simulink model "reaktor_m"  (R2016a)
settings: Solver=VariableStepAuto  StartTime=0.0  StopTime=400  RelTol=1e-3
undefined symbols (not defined in the file): AUXCO_0, B_t, C_0, linsys_matlab, P_cor0, ro_ex0, T_aves0, T_cl0, T_clp0, T_f10, T_f20, T_f30, T_hl0, T_hlp0, T_lp0, T_mo10, T_mo20, T_mo30, T_mo40, T_mo50, T_mo60, T_po0, T_set0, T_up0
settings Model: Creator=Użytkownik  LastModifiedBy=Michal Chruscinski
settings GRTTargetCC: GeneratePreprocessorConditionals=Use local settings

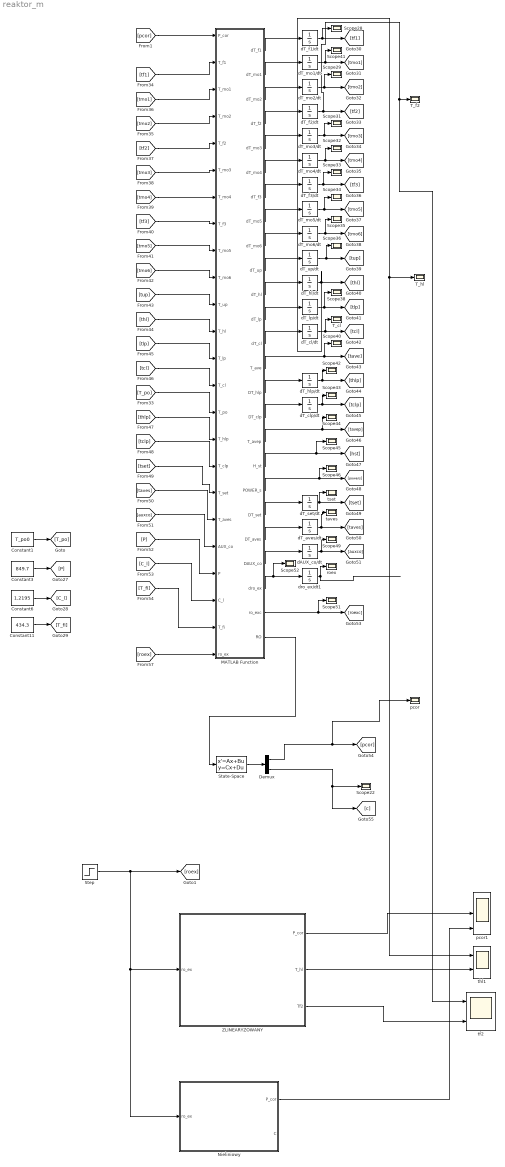
== system reaktor_m ==
  Constant1 : Constant  Value=T_po0
  Constant11 : Constant  Value=434.3
  Constant3 : Constant  Value=849.7
  Constant6 : Constant  Value=1.2195
  Demux : Demux  Outputs=2
  MATLAB Function : MATLAB Function  TreatAsAtomicUnit=on
  Nieliniowy : Subsystem
  Scope{22,28..29,31..36,38,40..46,49,51..52} (20 alike) : Scope
  State-Space : StateSpace  A=linsys_matlab.a  B=linsys_matlab.b  C=linsys_matlab.c  D=linsys_matlab.d  X0=0
  Step : Step  Time=0  After=0*B_t  SampleTime=0
  T_cl : Scope
  T_f2 : Scope
  T_hl : Scope
  ZLINEARYZOWANY : Subsystem
  dAUX_co/dt : Integrator  InitialCondition=AUXCO_0
  dT_aves/dt : Integrator  InitialCondition=T_aves0
  dT_cl/dt : Integrator  InitialCondition=T_cl0
  dT_clp/dt : Integrator  InitialCondition=T_clp0
  dT_f1/dt : Integrator  InitialCondition=T_f10
  dT_f2/dt : Integrator  InitialCondition=T_f20
  dT_f3/dt : Integrator  InitialCondition=T_f30
  dT_hl/dt : Integrator  InitialCondition=T_hl0
  dT_hlp/dt : Integrator  InitialCondition=T_hlp0
  dT_lp/dt : Integrator  InitialCondition=T_lp0
  dT_mo1/dt : Integrator  InitialCondition=T_mo10
  dT_mo2/dt : Integrator  InitialCondition=T_mo20
  dT_mo3/dt : Integrator  InitialCondition=T_mo30
  dT_mo4/dt : Integrator  InitialCondition=T_mo40
  dT_mo5/dt : Integrator  InitialCondition=T_mo50
  dT_mo6/dt : Integrator  InitialCondition=T_mo60
  dT_set/dt : Integrator  InitialCondition=T_set0
  dT_up/dt : Integrator  InitialCondition=T_up0
  dro_ex/dt1 : Integrator  InitialCondition=ro_ex0
  pcor : Scope
  pcor1 : Scope  NumInputPorts=3
  roex : Scope
  taves : Scope
  tf2 : Scope  NumInputPorts=2
  thl1 : Scope  NumInputPorts=2
  tset : Scope
  wires:
  Constant3/1 -> [P]
  Constant6/1 -> [C_l]
  Constant11/1 -> [T_fi]
  MATLAB Function/1(dT_f1) -> dT_f1/dt/1
  MATLAB Function/2(dT_mo1) -> dT_mo1/dt/1
  MATLAB Function/3(dT_mo2) -> dT_mo2/dt/1
  MATLAB Function/4(dT_f2) -> dT_f2/dt/1
  MATLAB Function/5(dT_mo3) -> dT_mo3/dt/1
  MATLAB Function/6(dT_mo4) -> dT_mo4/dt/1
  MATLAB Function/7(dT_f3) -> dT_f3/dt/1
  MATLAB Function/8(dT_mo5) -> dT_mo5/dt/1
  MATLAB Function/9(dT_mo6) -> dT_mo6/dt/1
  MATLAB Function/10(dT_up) -> dT_up/dt/1
  MATLAB Function/11(dT_hl) -> dT_hl/dt/1
  MATLAB Function/12(dT_lp) -> dT_lp/dt/1
  MATLAB Function/13(dT_cl) -> dT_cl/dt/1
  [T_po] -> MATLAB Function/15(T_po)
  dT_f1/dt/1 -> [tf1], Scope28/1
  dT_mo1/dt/1 -> Scope41/1, [tmo1]
  dT_mo2/dt/1 -> Scope29/1, [tmo2]
  dT_f2/dt/1 -> T_f2/1, tf2/1, [tf2]
  dT_mo3/dt/1 -> Scope31/1, [tmo3]
  dT_mo4/dt/1 -> Scope32/1, [tmo4]
  dT_f3/dt/1 -> Scope33/1, [tf3]
  dT_mo5/dt/1 -> Scope34/1, [tmo5]
  dT_mo6/dt/1 -> Scope35/1, [tmo6]
  dT_up/dt/1 -> Scope36/1, [tup]
  dT_hl/dt/1 -> [thl], thl1/1, T_hl/1
  dT_lp/dt/1 -> Scope38/1, [tlp]
  dT_cl/dt/1 -> T_cl/1, [tcl]
  [tf1] -> MATLAB Function/2(T_f1)
  [tmo2] -> MATLAB Function/4(T_mo2)
  [tmo1] -> MATLAB Function/3(T_mo1)
  [tf2] -> MATLAB Function/5(T_f2)
  [tmo3] -> MATLAB Function/6(T_mo3)
  [tmo4] -> MATLAB Function/7(T_mo4)
  [tf3] -> MATLAB Function/8(T_f3)
  [tmo5] -> MATLAB Function/9(T_mo5)
  [tmo6] -> MATLAB Function/10(T_mo6)
  [tup] -> MATLAB Function/11(T_up)
  [thl] -> MATLAB Function/12(T_hl)
  [tlp] -> MATLAB Function/13(T_lp)
  [tcl] -> MATLAB Function/14(T_cl)
  MATLAB Function/15(DT_hlp) -> dT_hlp/dt/1
  MATLAB Function/16(DT_clp) -> dT_clp/dt/1
  MATLAB Function/20(DT_set) -> dT_set/dt/1
  MATLAB Function/21(DT_aves) -> dT_aves/dt/1
  MATLAB Function/22(DAUX_co) -> dAUX_co/dt/1
  MATLAB Function/14(T_ave) -> Scope40/1, [tave]
  dT_hlp/dt/1 -> Scope42/1, [thlp]
  dT_clp/dt/1 -> Scope43/1, [tclp]
  MATLAB Function/17(T_avep) -> Scope44/1, [tavep]
  MATLAB Function/18(H_st) -> [hst], Scope45/1
  MATLAB Function/19(POWER_s) -> Scope46/1, [powers]
  dT_set/dt/1 -> tset/1, [tset]
  dT_aves/dt/1 -> [taves], taves/1
  dAUX_co/dt/1 -> [auxco], Scope49/1
  [thlp] -> MATLAB Function/16(T_hlp)
  [tclp] -> MATLAB Function/17(T_clp)
  [tset] -> MATLAB Function/18(T_set)
  [taves] -> MATLAB Function/19(T_aves)
  [auxco] -> MATLAB Function/20(AUX_co)
  [P] -> MATLAB Function/21(P)
  [C_l] -> MATLAB Function/22(C_l)
  [T_fi] -> MATLAB Function/23(T_fi)
  MATLAB Function/23(dro_ex) -> Scope52/1, dro_ex/dt1/1
  MATLAB Function/24(ro_exc) -> Scope51/1, [roexc]
  Constant1/1 -> [T_po]
  dro_ex/dt1/1 -> roex/1
  [roex] -> MATLAB Function/24(ro_ex)
  ZLINEARYZOWANY/1(P_cor) -> pcor1/2
  ZLINEARYZOWANY/2(T_hl) -> thl1/2
  ZLINEARYZOWANY/3(Tf2) -> tf2/2
  [pcor] -> MATLAB Function/1(P_cor)
  Demux/2 -> [c], Scope22/1
  Demux/1 -> [pcor], pcor/1
  MATLAB Function/25(RO) -> State-Space/1
  State-Space/1 -> Demux/1
  Nieliniowy/1(P_cor) -> pcor1/3
  Step/1 -> ZLINEARYZOWANY/1(ro_ex), Nieliniowy/1(ro_ex), [roex]

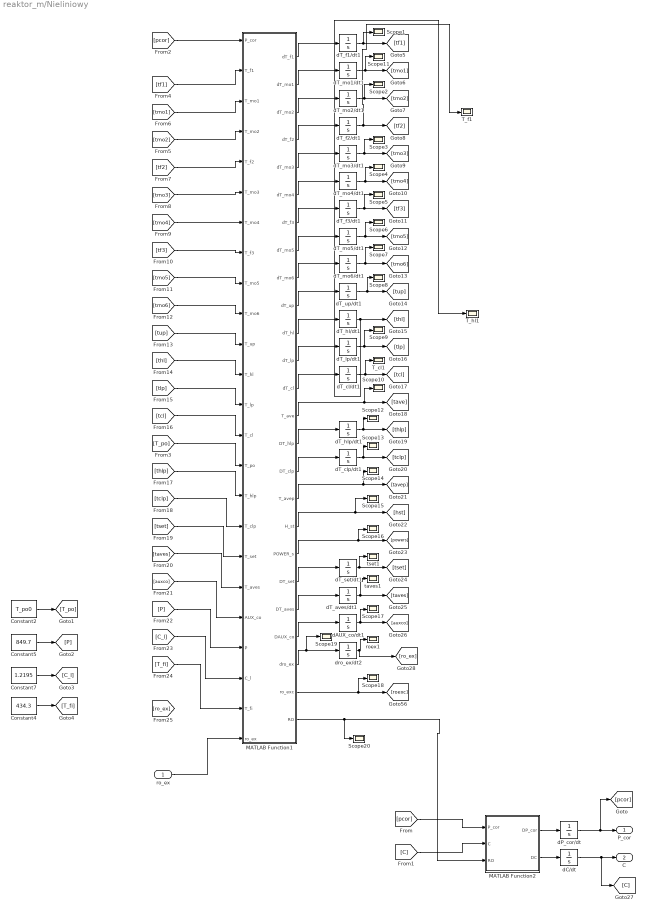
== system reaktor_m/Nieliniowy ==
  ro_ex : Inport
  Constant2 : Constant  Value=T_po0
  Constant4 : Constant  Value=434.3
  Constant5 : Constant  Value=849.7
  Constant7 : Constant  Value=1.2195
  MATLAB Function1 : MATLAB Function  TreatAsAtomicUnit=on
  MATLAB Function2 : MATLAB Function  TreatAsAtomicUnit=on
  Scope{1..20} (20 alike) : Scope
  T_cl1 : Scope
  T_f1 : Scope
  T_hl1 : Scope
  dAUX_co/dt1 : Integrator  InitialCondition=AUXCO_0
  dC/dt : Integrator  InitialCondition=C_0
  dP_cor/dt : Integrator  InitialCondition=P_cor0
  dT_aves/dt1 : Integrator  InitialCondition=T_aves0
  dT_cl/dt1 : Integrator  InitialCondition=T_cl0
  dT_clp/dt1 : Integrator  InitialCondition=T_clp0
  dT_f1/dt1 : Integrator  InitialCondition=T_f10
  dT_f2/dt1 : Integrator  InitialCondition=T_f20
  dT_f3/dt1 : Integrator  InitialCondition=T_f30
  dT_hl/dt1 : Integrator  InitialCondition=T_hl0
  dT_hlp/dt1 : Integrator  InitialCondition=T_hlp0
  dT_lp/dt1 : Integrator  InitialCondition=T_lp0
  dT_mo1/dt1 : Integrator  InitialCondition=T_mo10
  dT_mo2/dt1 : Integrator  InitialCondition=T_mo20
  dT_mo3/dt1 : Integrator  InitialCondition=T_mo30
  dT_mo4/dt1 : Integrator  InitialCondition=T_mo40
  dT_mo5/dt1 : Integrator  InitialCondition=T_mo50
  dT_mo6/dt1 : Integrator  InitialCondition=T_mo60
  dT_set/dt1 : Integrator  InitialCondition=T_set0
  dT_up/dt1 : Integrator  InitialCondition=T_up0
  dro_ex/dt2 : Integrator  InitialCondition=ro_ex0
  roex1 : Scope
  taves1 : Scope
  tset1 : Scope
  P_cor : Outport
  C : Outport  Port=2
  wires:
  dT_mo5/dt1/1 -> Scope6/1, [tmo5]
  MATLAB Function1/10(dT_up) -> dT_up/dt1/1
  [T_po] -> MATLAB Function1/15(T_po)
  dT_mo6/dt1/1 -> Scope7/1, [tmo6]
  dT_lp/dt1/1 -> Scope9/1, [tlp]
  Constant5/1 -> [P]
  Constant7/1 -> [C_l]
  Constant4/1 -> [T_fi]
  MATLAB Function1/8(dT_mo5) -> dT_mo5/dt1/1
  MATLAB Function1/2(dT_mo1) -> dT_mo1/dt1/1
  MATLAB Function1/5(dT_mo3) -> dT_mo3/dt1/1
  MATLAB Function1/3(dT_mo2) -> dT_mo2/dt1/1
  dT_f2/dt1/1 -> T_f1/1, [tf2]
  dT_mo4/dt1/1 -> Scope4/1, [tmo4]
  dT_f3/dt1/1 -> Scope5/1, [tf3]
  MATLAB Function1/1(dT_f1) -> dT_f1/dt1/1
  dT_hl/dt1/1 -> [thl], T_hl1/1
  dT_cl/dt1/1 -> T_cl1/1, [tcl]
  MATLAB Function1/7(dT_f3) -> dT_f3/dt1/1
  dT_f1/dt1/1 -> [tf1], Scope1/1
  dT_mo1/dt1/1 -> Scope11/1, [tmo1]
  MATLAB Function1/11(dT_hl) -> dT_hl/dt1/1
  dT_mo3/dt1/1 -> Scope3/1, [tmo3]
  MATLAB Function1/6(dT_mo4) -> dT_mo4/dt1/1
  MATLAB Function1/9(dT_mo6) -> dT_mo6/dt1/1
  dT_up/dt1/1 -> Scope8/1, [tup]
  MATLAB Function1/4(dT_f2) -> dT_f2/dt1/1
  MATLAB Function1/12(dT_lp) -> dT_lp/dt1/1
  dT_mo2/dt1/1 -> Scope2/1, [tmo2]
  MATLAB Function1/13(dT_cl) -> dT_cl/dt1/1
  dT_set/dt1/1 -> tset1/1, [tset]
  MATLAB Function1/16(DT_clp) -> dT_clp/dt1/1
  [tmo3] -> MATLAB Function1/6(T_mo3)
  dT_hlp/dt1/1 -> Scope12/1, [thlp]
  [tmo6] -> MATLAB Function1/10(T_mo6)
  MATLAB Function1/15(DT_hlp) -> dT_hlp/dt1/1
  dro_ex/dt2/1 -> [ro_ex], roex1/1
  [thl] -> MATLAB Function1/12(T_hl)
  dT_clp/dt1/1 -> Scope13/1, [tclp]
  [auxco] -> MATLAB Function1/20(AUX_co)
  [tmo1] -> MATLAB Function1/3(T_mo1)
  [tclp] -> MATLAB Function1/17(T_clp)
  [pcor] -> MATLAB Function1/1(P_cor)
  MATLAB Function1/18(H_st) -> [hst], Scope15/1
  MATLAB Function1/20(DT_set) -> dT_set/dt1/1
  MATLAB Function1/17(T_avep) -> Scope14/1, [tavep]
  [tf2] -> MATLAB Function1/5(T_f2)
  MATLAB Function1/19(POWER_s) -> Scope16/1, [powers]
  [tf1] -> MATLAB Function1/2(T_f1)
  MATLAB Function1/14(T_ave) -> Scope10/1, [tave]
  dT_aves/dt1/1 -> [taves], taves1/1
  [tlp] -> MATLAB Function1/13(T_lp)
  dAUX_co/dt1/1 -> [auxco], Scope17/1
  [tup] -> MATLAB Function1/11(T_up)
  [tmo5] -> MATLAB Function1/9(T_mo5)
  [taves] -> MATLAB Function1/19(T_aves)
  [P] -> MATLAB Function1/21(P)
  [tf3] -> MATLAB Function1/8(T_f3)
  MATLAB Function1/21(DT_aves) -> dT_aves/dt1/1
  [tcl] -> MATLAB Function1/14(T_cl)
  [C_l] -> MATLAB Function1/22(C_l)
  [T_fi] -> MATLAB Function1/23(T_fi)
  [tmo2] -> MATLAB Function1/4(T_mo2)
  MATLAB Function1/22(DAUX_co) -> dAUX_co/dt1/1
  [tset] -> MATLAB Function1/18(T_set)
  MATLAB Function1/23(dro_ex) -> Scope19/1, dro_ex/dt2/1
  [tmo4] -> MATLAB Function1/7(T_mo4)
  Constant2/1 -> [T_po]
  [thlp] -> MATLAB Function1/16(T_hlp)
  MATLAB Function1/24(ro_exc) -> Scope18/1, [roexc]
  MATLAB Function2/2(DC) -> dC/dt/1
  MATLAB Function2/1(DP_cor) -> dP_cor/dt/1
  dP_cor/dt/1 -> [pcor], P_cor/1
  dC/dt/1 -> [C], C/1
  MATLAB Function1/25(RO) -> Scope20/1, MATLAB Function2/3(RO)
  [pcor] -> MATLAB Function2/1(P_cor)
  [C] -> MATLAB Function2/2(C)
  ro_ex/1 -> MATLAB Function1/24(ro_ex)

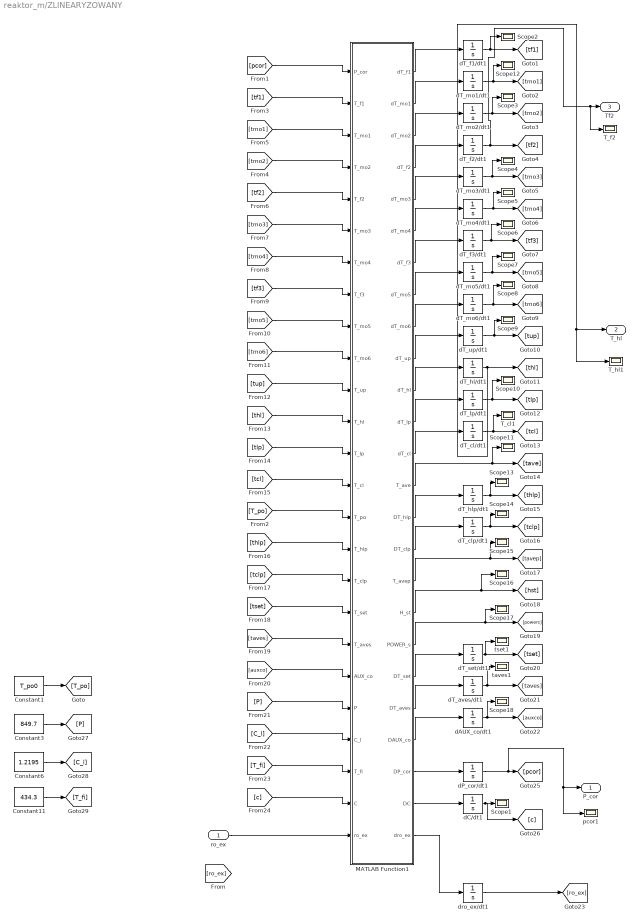
== system reaktor_m/ZLINEARYZOWANY ==
  ro_ex : Inport
  Constant1 : Constant  Value=T_po0
  Constant11 : Constant  Value=434.3
  Constant3 : Constant  Value=849.7
  Constant6 : Constant  Value=1.2195
  MATLAB Function1 : MATLAB Function  TreatAsAtomicUnit=on
  Scope{1..18} (18 alike) : Scope
  T_cl1 : Scope
  T_f2 : Scope
  T_hl1 : Scope
  dAUX_co/dt1 : Integrator  InitialCondition=AUXCO_0
  dC/dt1 : Integrator  InitialCondition=C_0
  dP_cor/dt1 : Integrator  InitialCondition=P_cor0
  dT_aves/dt1 : Integrator  InitialCondition=T_aves0
  dT_cl/dt1 : Integrator  InitialCondition=T_cl0
  dT_clp/dt1 : Integrator  InitialCondition=T_clp0
  dT_f1/dt1 : Integrator  InitialCondition=T_f10
  dT_f2/dt1 : Integrator  InitialCondition=T_f20
  dT_f3/dt1 : Integrator  InitialCondition=T_f30
  dT_hl/dt1 : Integrator  InitialCondition=T_hl0
  dT_hlp/dt1 : Integrator  InitialCondition=T_hlp0
  dT_lp/dt1 : Integrator  InitialCondition=T_lp0
  dT_mo1/dt1 : Integrator  InitialCondition=T_mo10
  dT_mo2/dt1 : Integrator  InitialCondition=T_mo20
  dT_mo3/dt1 : Integrator  InitialCondition=T_mo30
  dT_mo4/dt1 : Integrator  InitialCondition=T_mo40
  dT_mo5/dt1 : Integrator  InitialCondition=T_mo50
  dT_mo6/dt1 : Integrator  InitialCondition=T_mo60
  dT_set/dt1 : Integrator  InitialCondition=T_set0
  dT_up/dt1 : Integrator  InitialCondition=T_up0
  dro_ex/dt1 : Integrator  InitialCondition=ro_ex0
  pcor1 : Scope
  taves1 : Scope
  tset1 : Scope
  P_cor : Outport
  T_hl : Outport  Port=2
  Tf2 : Outport  Port=3
  wires:
  dT_f2/dt1/1 -> Tf2/1, T_f2/1, [tf2]
  dT_up/dt1/1 -> Scope9/1, [tup]
  [pcor] -> MATLAB Function1/1(P_cor)
  MATLAB Function1/10(dT_up) -> dT_up/dt1/1
  dT_mo1/dt1/1 -> Scope12/1, [tmo1]
  MATLAB Function1/5(dT_mo3) -> dT_mo3/dt1/1
  MATLAB Function1/9(dT_mo6) -> dT_mo6/dt1/1
  dT_mo2/dt1/1 -> Scope3/1, [tmo2]
  dT_mo3/dt1/1 -> Scope4/1, [tmo3]
  MATLAB Function1/11(dT_hl) -> dT_hl/dt1/1
  dT_mo6/dt1/1 -> Scope8/1, [tmo6]
  dT_f3/dt1/1 -> Scope6/1, [tf3]
  dT_f1/dt1/1 -> [tf1], Scope2/1
  dT_hl/dt1/1 -> [thl], T_hl/1, T_hl1/1
  MATLAB Function1/2(dT_mo1) -> dT_mo1/dt1/1
  MATLAB Function1/1(dT_f1) -> dT_f1/dt1/1
  MATLAB Function1/3(dT_mo2) -> dT_mo2/dt1/1
  MATLAB Function1/4(dT_f2) -> dT_f2/dt1/1
  [T_po] -> MATLAB Function1/15(T_po)
  dT_mo4/dt1/1 -> Scope5/1, [tmo4]
  dT_mo5/dt1/1 -> Scope7/1, [tmo5]
  dT_lp/dt1/1 -> Scope10/1, [tlp]
  MATLAB Function1/6(dT_mo4) -> dT_mo4/dt1/1
  dT_cl/dt1/1 -> T_cl1/1, [tcl]
  MATLAB Function1/7(dT_f3) -> dT_f3/dt1/1
  MATLAB Function1/8(dT_mo5) -> dT_mo5/dt1/1
  MATLAB Function1/12(dT_lp) -> dT_lp/dt1/1
  MATLAB Function1/13(dT_cl) -> dT_cl/dt1/1
  dT_set/dt1/1 -> tset1/1, [tset]
  dAUX_co/dt1/1 -> [auxco], Scope18/1
  [tclp] -> MATLAB Function1/17(T_clp)
  [thl] -> MATLAB Function1/12(T_hl)
  dT_aves/dt1/1 -> [taves], taves1/1
  dT_clp/dt1/1 -> Scope14/1, [tclp]
  [thlp] -> MATLAB Function1/16(T_hlp)
  dP_cor/dt1/1 -> P_cor/1, pcor1/1, [pcor]
  MATLAB Function1/15(DT_hlp) -> dT_hlp/dt1/1
  MATLAB Function1/18(H_st) -> [hst], Scope16/1
  [T_fi] -> MATLAB Function1/23(T_fi)
  MATLAB Function1/22(DAUX_co) -> dAUX_co/dt1/1
  [tmo2] -> MATLAB Function1/4(T_mo2)
  [c] -> MATLAB Function1/24(C)
  [P] -> MATLAB Function1/21(P)
  [auxco] -> MATLAB Function1/20(AUX_co)
  [tlp] -> MATLAB Function1/13(T_lp)
  [tcl] -> MATLAB Function1/14(T_cl)
  MATLAB Function1/16(DT_clp) -> dT_clp/dt1/1
  MATLAB Function1/14(T_ave) -> Scope11/1, [tave]
  [tf3] -> MATLAB Function1/8(T_f3)
  MATLAB Function1/20(DT_set) -> dT_set/dt1/1
  [tup] -> MATLAB Function1/11(T_up)
  dT_hlp/dt1/1 -> Scope13/1, [thlp]
  MATLAB Function1/19(POWER_s) -> Scope17/1, [powers]
  [tset] -> MATLAB Function1/18(T_set)
  [tmo3] -> MATLAB Function1/6(T_mo3)
  MATLAB Function1/24(DC) -> dC/dt1/1
  [tmo6] -> MATLAB Function1/10(T_mo6)
  dC/dt1/1 -> [c], Scope1/1
  [taves] -> MATLAB Function1/19(T_aves)
  [C_l] -> MATLAB Function1/22(C_l)
  MATLAB Function1/23(DP_cor) -> dP_cor/dt1/1
  [tmo1] -> MATLAB Function1/3(T_mo1)
  [tf2] -> MATLAB Function1/5(T_f2)
  MATLAB Function1/21(DT_aves) -> dT_aves/dt1/1
  MATLAB Function1/17(T_avep) -> Scope15/1, [tavep]
  [tmo4] -> MATLAB Function1/7(T_mo4)
  [tf1] -> MATLAB Function1/2(T_f1)
  [tmo5] -> MATLAB Function1/9(T_mo5)
  Constant3/1 -> [P]
  Constant6/1 -> [C_l]
  Constant11/1 -> [T_fi]
  Constant1/1 -> [T_po]
  MATLAB Function1/25(dro_ex) -> dro_ex/dt1/1
  dro_ex/dt1/1 -> [ro_ex]
  ro_ex/1 -> MATLAB Function1/25(ro_ex)

== matlab function reaktor_m/ZLINEARYZOWANY/MATLAB Function1 ==
  data: P_cor input; T_f1 input; T_mo1 input; T_mo2 input; T_f2 input; T_mo3 input; T_mo4 input; T_f3 input; T_mo5 input; T_mo6 input; T_up input; T_hl input; dT_f1 output; dT_mo1 output; dT_mo2 output; dT_f2 output; dT_mo3 output; dT_mo4 output; dT_f3 output; dT_mo5 output; dT_mo6 output; T_lp input; T_cl input; dT_up output; dT_hl output; dT_lp output; dT_cl output; T_po input; T_hlp input; T_clp input; T_set input; T_aves input; AUX_co input; T_ave output; DT_hlp output; DT_clp output; T_avep output; H_st output; POWER_s output; DT_set output; DT_aves output; DAUX_co output; P input; C_l input; T_fi input; DP_cor output; DC output; C input; ro_ex input; dro_ex output
function [dT_f1,dT_mo1,dT_mo2,dT_f2,dT_mo3,dT_mo4,dT_f3,dT_mo5,dT_mo6,dT_up,dT_hl,dT_lp,dT_cl,T_ave,DT_hlp,DT_clp,T_avep,H_st,POWER_s,DT_set,DT_aves,DAUX_co,DP_cor,DC,dro_ex] = fcn(P_cor,T_f1,T_mo1,T_mo2,T_f2,T_mo3,T_mo4,T_f3,T_mo5,T_mo6,T_up,T_hl,T_lp,T_cl,T_po,T_hlp,T_clp,T_set,T_aves,AUX_co,P,C_l,T_fi,C,ro_ex)
%#codegen

%%%%%%%%%%%%%%%% STAŁE

M_ft = 222739;
C_pf = 0.059;
C_pf = 0.059;
C_pmo = 1.39;
F_r = 0.974;
P_cor0 = 1;
ro0 = 3e-7;
C0 = 4625.71;


%%%%%%%% OBLICZANIE STALYCH WIELKOSCI

P_cor10 = 3.436 * 10^9;
W_pth = 1.57559 * 10^8;
V_up = 1376;
V_lp = 1791;
V_hl = 1000;
V_cl = 2000;
V_mo = 540;
DENS_mo = 45.71;
C_pmo = 1.39;

P_cor1 = (P_cor10 * 3.41) / (3600 * 3);
H_fm= 200/3600;
A_fm = 59900/3;
W_pt = W_pth/3600;

M_f = M_ft * 3;
M_mo = V_mo * DENS_mo / 3;
M_up = V_up * DENS_mo;
M_lp = V_lp * DENS_mo;
M_hl = V_hl * DENS_mo;
M_cl = V_cl * DENS_mo;

tau_mo = M_mo / (2 * W_pt);
tau_up = M_up / W_pt;
tau_lp = M_lp / W_pt;
tau_hl = M_hl / W_pt;
tau_cl = M_cl / W_pt;

%%%%% OBLICZENIA DLA POCHODNYCH MODELU REAKTORA

DT_f1 = (F_r*P_cor1*P_cor) / (M_f*C_pf) + (H_fm*A_fm)*(T_mo1 -T_f1) / (M_f*C_pf);
DT_mo1 = ( (1 -F_r)*P_cor1*P_cor ) / (M_mo*C_pmo) + (H_fm*A_fm)*(T_f1-T_mo1) / (M_mo*C_pmo) + (T_lp-T_mo1) / tau_mo;
DT_mo2 = ( (1 -F_r)*P_cor1*P_cor ) / (M_mo*C_pmo) + (H_fm*A_fm)*(T_f1-T_mo1) / (M_mo*C_pmo) + (T_mo1-T_mo2) / tau_mo;

DT_f2 = (F_r*P_cor1*P_cor) / (M_f*C_pf) + (H_fm*A_fm)*(T_mo3-T_f2) / (M_f*C_pf);
DT_mo3 = ( (1-F_r)*P_cor1*P_cor ) / (M_mo*C_pmo) + (H_fm*A_fm)*(T_f2-T_mo3) / (M_mo*C_pmo) + (T_mo2-T_mo3) / tau_mo;
DT_mo4 = ( (1-F_r)*P_cor1*P_cor ) / (M_mo*C_pmo) + (H_fm*A_fm)*(T_f2-T_mo3) / (M_mo*C_pmo) + (T_mo3-T_mo4) / tau_mo;

DT_f3 = (F_r*P_cor1*P_cor) / (M_f*C_pf) + (H_fm*A_fm)*(T_mo5-T_f3) / (M_f *C_pf);
DT_mo5 = ( (1-F_r)*P_cor1*P_cor) / (M_mo*C_pmo) + (H_fm*A_fm) * (T_f3-T_mo5) / (M_mo*C_pmo) + (T_mo4-T_mo5) / tau_mo;
DT_mo6 = ( (1-F_r)*P_cor1*P_cor) / (M_mo*C_pmo) + (H_fm*A_fm) * (T_f3-T_mo5) / (M_mo*C_pmo) + (T_mo5-T_mo6) / tau_mo;

DT_up = (T_mo6-T_up) / tau_up;
DT_hl = (T_up-T_hl) / tau_hl;
DT_lp = (T_cl-T_lp) / tau_lp;
DT_cl = (T_po-T_cl) / tau_cl;


%%%%%% OBLICZENIA DO KONTROLI SYSTEMU REAKTORA
%%%%%zmienne które jeszcze sa wejsciem P,CL,T_fi
POWER_i = 691244.4199;
tau_set = 30;
tau_la1 = 10;
tau_la2 = 5;
tau_le = 80;
tau_rtd = 4;
C_pfw = 1.2181;
K9 = -0.035;
X8 = 1225.85;

T_ave = (T_cl+T_hl) / 2;
DT_hlp = (T_hl-T_hlp) / tau_rtd;
DT_clp = (T_cl-T_clp) / tau_rtd;
T_avep = (T_hlp+T_clp) / 2;

H_st = X8 + (K9*P);
POWER_s= P*C_l*( H_st - (C_pfw*T_fi) );

DT_set = ( 0.19*(POWER_s*100 / POWER_i) + 547 - T_set ) /tau_set;
DT_aves = AUX_co;
DAUX_co = ( T_avep - T_aves - (tau_la1+tau_la2)*AUX_co + tau_le*(DT_clp+DT_hlp) /2 ) / (tau_la1*tau_la2);
 
%%%%%%%%%%%%%%%%%%%%%%%%%%% REAKTOR

BETA1 = 0.000209;
BETA2 = 0.001414;
BETA3 = 0.001309;
BETA4 = 0.002727;
BETA5 = 0.000925;
BETA6 = 0.000314;

BETA_t =  0.00689;

LANDA1 = 0.0125;
LANDA2 = 0.0308;
LANDA3 = 0.114;
LANDA4 = 0.307;
LANDA5 = 1.19;
LANDA6 = 3.19;

T_f10 = 1488.75;
T_mo10 = 548.303;
T_mo20 = 557.106;
T_f20 = 1506.38;
T_mo30 = 565.909;
T_mo40 = 574.711;
T_f30 = 1523.96;
T_mo50 = 583.514;
T_mo60 = 592.5;

alfa_f = -1.1 * 10^-5;

alfa_c = -2.0 * 10^-4;

NGT = 17.9 * 10^-6;

LANDA = BETA_t / (BETA1/LANDA1 + BETA2/LANDA2 + BETA3/LANDA3 + BETA4/LANDA4 + BETA5/LANDA5 + BETA6/LANDA6);

RO = ro_ex + alfa_f *( (T_f1-T_f10) + (T_f2-T_f20) + (T_f3-T_f30) ) /3 + alfa_c* ( (T_mo1-T_mo10) + (T_mo2-T_mo20)+ (T_mo3 -T_mo30) + (T_mo4-T_mo40 ) + (T_mo5-T_mo50) + (T_mo6-T_mo60) ) /6;

DC = BETA_t*P_cor / NGT - LANDA*C;
 
%%%%% ZLINEARYZOWANY P_cor
delta_P_cor = P_cor - P_cor0;
delta_ro = RO - ro0;
delta_C = C - C0;
DP_cor = ((ro0-BETA_t)/NGT)*delta_P_cor + (P_cor0/NGT)*delta_ro + LANDA*delta_C;
 
%%%%%% STEROWANIE REAKTOREM



e = T_set - T_aves;

React = 0.003375;

 if e >= 5
     dro_ex = (72 * React * 0.00689) / 60;
 elseif e < 5 && e >= 3 
     dro_ex = (React * 0.00689 * (32 * (T_set-T_aves) - 88)) / 60;
 elseif e < 3 && e >= 1 
     dro_ex = (8 * React * 0.00689) / 60;
 elseif abs(e) < 1
     dro_ex = 0;
 elseif e <= -1 && e >= -3 
     dro_ex = (-8 * React * 0.00689) / 60;
 elseif e < -3 && e >= -5
     dro_ex = (React * 0.00689 * (32 * (T_set-T_aves) + 88)) / 60;
 else
     dro_ex = (-72 * React * 0.00689) / 60;
 end

%%%%% ZMIENNE WYJŚCIOWE

dT_f1 = DT_f1;
dT_mo1 = DT_mo1;
dT_mo2 = DT_mo2;
dT_f2 = DT_f2;
dT_mo3 = DT_mo3;
dT_mo4 = DT_mo4;
dT_f3 = DT_f3;
dT_mo5 = DT_mo5;
dT_mo6 = DT_mo6;

dT_up = DT_up;
dT_hl = DT_hl;
dT_lp = DT_lp;
dT_cl = DT_cl;

== matlab function reaktor_m/Nieliniowy/MATLAB Function2 ==
  data: P_cor input; DP_cor output; DC output; C input; RO input
function [DP_cor,DC] = fcn(P_cor,C,RO)
%#codegen
%%%%%%%%%%%%%%%%%%%%%%%%%%% REAKTOR

BETA1 = 0.000209;
BETA2 = 0.001414;
BETA3 = 0.001309;
BETA4 = 0.002727;
BETA5 = 0.000925;
BETA6 = 0.000314;

BETA_t =  0.00689;

LANDA1 = 0.0125;
LANDA2 = 0.0308;
LANDA3 = 0.114;
LANDA4 = 0.307;
LANDA5 = 1.19;
LANDA6 = 3.19;

NGT = 17.9 * 10^-6;

LANDA = BETA_t / (BETA1/LANDA1 + BETA2/LANDA2 + BETA3/LANDA3 + BETA4/LANDA4 + BETA5/LANDA5 + BETA6/LANDA6);

DP_cor = (RO-BETA_t)*P_cor / NGT + LANDA*C;
DC = BETA_t*P_cor / NGT - LANDA*C;

== matlab function reaktor_m/MATLAB Function ==
  data: P_cor input; T_f1 input; T_mo1 input; T_mo2 input; T_f2 input; T_mo3 input; T_mo4 input; T_f3 input; T_mo5 input; T_mo6 input; T_up input; T_hl input; dT_f1 output; dT_mo1 output; dT_mo2 output; dT_f2 output; dT_mo3 output; dT_mo4 output; dT_f3 output; dT_mo5 output; dT_mo6 output; T_lp input; T_cl input; dT_up output; dT_hl output; dT_lp output; dT_cl output; T_po input; T_hlp input; T_clp input; T_set input; T_aves input; AUX_co input; T_ave output; DT_hlp output; DT_clp output; T_avep output; H_st output; POWER_s output; DT_set output; DT_aves output; DAUX_co output; P input; C_l input; T_fi input; dro_ex output; ro_exc output; ro_ex input; RO output
function [dT_f1,dT_mo1,dT_mo2,dT_f2,dT_mo3,dT_mo4,dT_f3,dT_mo5,dT_mo6,dT_up,dT_hl,dT_lp,dT_cl,T_ave,DT_hlp,DT_clp,T_avep,H_st,POWER_s,DT_set,DT_aves,DAUX_co,dro_ex,ro_exc,RO] = fcn(P_cor,T_f1,T_mo1,T_mo2,T_f2,T_mo3,T_mo4,T_f3,T_mo5,T_mo6,T_up,T_hl,T_lp,T_cl,T_po,T_hlp,T_clp,T_set,T_aves,AUX_co,P,C_l,T_fi,ro_ex)
%#codegen

%%%%%%%%%%%%%%%% STAŁE

M_ft = 222739;
C_pf = 0.059;
C_pf = 0.059;
C_pmo = 1.39;
F_r = 0.974;


%%%%%%%% OBLICZANIE STALYCH WIELKOSCI

P_cor10 = 3.436 * 10^9;
W_pth = 1.57559 * 10^8;
V_up = 1376;
V_lp = 1791;
V_hl = 1000;
V_cl = 2000;
V_mo = 540;
DENS_mo = 45.71;
C_pmo = 1.39;

P_cor1 = (P_cor10 * 3.41) / (3600 * 3);
H_fm= 200/3600;
A_fm = 59900/3;
W_pt = W_pth/3600;

M_f = M_ft * 3;
M_mo = V_mo * DENS_mo / 3;
M_up = V_up * DENS_mo;
M_lp = V_lp * DENS_mo;
M_hl = V_hl * DENS_mo;
M_cl = V_cl * DENS_mo;

tau_mo = M_mo / (2 * W_pt);
tau_up = M_up / W_pt;
tau_lp = M_lp / W_pt;
tau_hl = M_hl / W_pt;
tau_cl = M_cl / W_pt;

%%%%% OBLICZENIA DLA POCHODNYCH MODELU REAKTORA

DT_f1 = (F_r*P_cor1*P_cor) / (M_f*C_pf) + (H_fm*A_fm)*(T_mo1 -T_f1) / (M_f*C_pf);
DT_mo1 = ( (1 -F_r)*P_cor1*P_cor ) / (M_mo*C_pmo) + (H_fm*A_fm)*(T_f1-T_mo1) / (M_mo*C_pmo) + (T_lp-T_mo1) / tau_mo;
DT_mo2 = ( (1 -F_r)*P_cor1*P_cor ) / (M_mo*C_pmo) + (H_fm*A_fm)*(T_f1-T_mo1) / (M_mo*C_pmo) + (T_mo1-T_mo2) / tau_mo;

DT_f2 = (F_r*P_cor1*P_cor) / (M_f*C_pf) + (H_fm*A_fm)*(T_mo3-T_f2) / (M_f*C_pf);
DT_mo3 = ( (1-F_r)*P_cor1*P_cor ) / (M_mo*C_pmo) + (H_fm*A_fm)*(T_f2-T_mo3) / (M_mo*C_pmo) + (T_mo2-T_mo3) / tau_mo;
DT_mo4 = ( (1-F_r)*P_cor1*P_cor ) / (M_mo*C_pmo) + (H_fm*A_fm)*(T_f2-T_mo3) / (M_mo*C_pmo) + (T_mo3-T_mo4) / tau_mo;

DT_f3 = (F_r*P_cor1*P_cor) / (M_f*C_pf) + (H_fm*A_fm)*(T_mo5-T_f3) / (M_f *C_pf);
DT_mo5 = ( (1-F_r)*P_cor1*P_cor) / (M_mo*C_pmo) + (H_fm*A_fm) * (T_f3-T_mo5) / (M_mo*C_pmo) + (T_mo4-T_mo5) / tau_mo;
DT_mo6 = ( (1-F_r)*P_cor1*P_cor) / (M_mo*C_pmo) + (H_fm*A_fm) * (T_f3-T_mo5) / (M_mo*C_pmo) + (T_mo5-T_mo6) / tau_mo;

DT_up = (T_mo6-T_up) / tau_up;
DT_hl = (T_up-T_hl) / tau_hl;
DT_lp = (T_cl-T_lp) / tau_lp;
DT_cl = (T_po-T_cl) / tau_cl;


%%%%%% OBLICZENIA DO KONTROLI SYSTEMU REAKTORA
%%%%%zmienne które jeszcze sa wejsciem P,CL,T_fi
POWER_i = 691244.4199;
tau_set = 30;
tau_la1 = 10;
tau_la2 = 5;
tau_le = 80;
tau_rtd = 4;
C_pfw = 1.2181;
K9 = -0.035;
X8 = 1225.85;

T_ave = (T_cl+T_hl) / 2;
DT_hlp = (T_hl-T_hlp) / tau_rtd;
DT_clp = (T_cl-T_clp) / tau_rtd;
T_avep = (T_hlp+T_clp) / 2;

H_st = X8 + (K9*P);
POWER_s= P*C_l*( H_st - (C_pfw*T_fi) );

DT_set = ( 0.19*(POWER_s*100 / POWER_i) + 547 - T_set ) /tau_set;
DT_aves = AUX_co;
DAUX_co = ( T_avep - T_aves - (tau_la1+tau_la2)*AUX_co + tau_le*(DT_clp+DT_hlp) /2 ) / (tau_la1*tau_la2);

%%%%%% STEROWANIE REAKTOREM



e = T_set - T_aves;

React = 0.003375;

 if e >= 5
     dro_ex = (72 * React * 0.00689) / 60;
 elseif e < 5 && e >= 3 
     dro_ex = (React * 0.00689 * (32 * (T_set-T_aves) - 88)) / 60;
 elseif e < 3 && e >= 1 
     dro_ex = (8 * React * 0.00689) / 60;
 elseif abs(e) < 1
     dro_ex = 0;
 elseif e <= -1 && e >= -3 
     dro_ex = (-8 * React * 0.00689) / 60;
 elseif e < -3 && e >= -5
     dro_ex = (React * 0.00689 * (32 * (T_set-T_aves) + 88)) / 60;
 else
     dro_ex = (-72 * React * 0.00689) / 60;
 end
 
 ro_exc= ro_ex*100 / 0.00689 ;
 
%%%%%%%%%%%%%%%%%%%%%%%%%%% REAKTOR

T_f10 = 1488.75;
T_mo10 = 548.303;
T_mo20 = 557.106;
T_f20 = 1506.38;
T_mo30 = 565.909;
T_mo40 = 574.711;
T_f30 = 1523.96;
T_mo50 = 583.514;
T_mo60 = 592.5;

alfa_f = -1.1 * 10^-5;

alfa_c = -2.0 * 10^-4;

RO = ro_ex + alfa_f *( (T_f1-T_f10) + (T_f2-T_f20) + (T_f3-T_f30) ) /3 + alfa_c* ( (T_mo1-T_mo10) + (T_mo2-T_mo20)+ (T_mo3 -T_mo30) + (T_mo4-T_mo40 ) + (T_mo5-T_mo50) + (T_mo6-T_mo60) ) /6;
 
%%%%% ZMIENNE WYJŚCIOWE

dT_f1 = DT_f1;
dT_mo1 = DT_mo1;
dT_mo2 = DT_mo2;
dT_f2 = DT_f2;
dT_mo3 = DT_mo3;
dT_mo4 = DT_mo4;
dT_f3 = DT_f3;
dT_mo5 = DT_mo5;
dT_mo6 = DT_mo6;

dT_up = DT_up;
dT_hl = DT_hl;
dT_lp = DT_lp;
dT_cl = DT_cl;

== matlab function reaktor_m/Nieliniowy/MATLAB Function1 ==
  data: P_cor input; T_f1 input; T_mo1 input; T_mo2 input; T_f2 input; T_mo3 input; T_mo4 input; T_f3 input; T_mo5 input; T_mo6 input; T_up input; T_hl input; dT_f1 output; dT_mo1 output; dT_mo2 output; dT_f2 output; dT_mo3 output; dT_mo4 output; dT_f3 output; dT_mo5 output; dT_mo6 output; T_lp input; T_cl input; dT_up output; dT_hl output; dT_lp output; dT_cl output; T_po input; T_hlp input; T_clp input; T_set input; T_aves input; AUX_co input; T_ave output; DT_hlp output; DT_clp output; T_avep output; H_st output; POWER_s output; DT_set output; DT_aves output; DAUX_co output; P input; C_l input; T_fi input; dro_ex output; ro_exc output; ro_ex input; RO output
function [dT_f1,dT_mo1,dT_mo2,dT_f2,dT_mo3,dT_mo4,dT_f3,dT_mo5,dT_mo6,dT_up,dT_hl,dT_lp,dT_cl,T_ave,DT_hlp,DT_clp,T_avep,H_st,POWER_s,DT_set,DT_aves,DAUX_co,dro_ex,ro_exc,RO] = fcn(P_cor,T_f1,T_mo1,T_mo2,T_f2,T_mo3,T_mo4,T_f3,T_mo5,T_mo6,T_up,T_hl,T_lp,T_cl,T_po,T_hlp,T_clp,T_set,T_aves,AUX_co,P,C_l,T_fi,ro_ex)
%#codegen

%%%%%%%%%%%%%%%% STAŁE

M_ft = 222739;
C_pf = 0.059;
C_pf = 0.059;
C_pmo = 1.39;
F_r = 0.974;


%%%%%%%% OBLICZANIE STALYCH WIELKOSCI

P_cor10 = 3.436 * 10^9;
W_pth = 1.57559 * 10^8;
V_up = 1376;
V_lp = 1791;
V_hl = 1000;
V_cl = 2000;
V_mo = 540;
DENS_mo = 45.71;
C_pmo = 1.39;

P_cor1 = (P_cor10 * 3.41) / (3600 * 3);
H_fm= 200/3600;
A_fm = 59900/3;
W_pt = W_pth/3600;

M_f = M_ft * 3;
M_mo = V_mo * DENS_mo / 3;
M_up = V_up * DENS_mo;
M_lp = V_lp * DENS_mo;
M_hl = V_hl * DENS_mo;
M_cl = V_cl * DENS_mo;

tau_mo = M_mo / (2 * W_pt);
tau_up = M_up / W_pt;
tau_lp = M_lp / W_pt;
tau_hl = M_hl / W_pt;
tau_cl = M_cl / W_pt;

%%%%% OBLICZENIA DLA POCHODNYCH MODELU REAKTORA

DT_f1 = (F_r*P_cor1*P_cor) / (M_f*C_pf) + (H_fm*A_fm)*(T_mo1 -T_f1) / (M_f*C_pf);
DT_mo1 = ( (1 -F_r)*P_cor1*P_cor ) / (M_mo*C_pmo) + (H_fm*A_fm)*(T_f1-T_mo1) / (M_mo*C_pmo) + (T_lp-T_mo1) / tau_mo;
DT_mo2 = ( (1 -F_r)*P_cor1*P_cor ) / (M_mo*C_pmo) + (H_fm*A_fm)*(T_f1-T_mo1) / (M_mo*C_pmo) + (T_mo1-T_mo2) / tau_mo;

DT_f2 = (F_r*P_cor1*P_cor) / (M_f*C_pf) + (H_fm*A_fm)*(T_mo3-T_f2) / (M_f*C_pf);
DT_mo3 = ( (1-F_r)*P_cor1*P_cor ) / (M_mo*C_pmo) + (H_fm*A_fm)*(T_f2-T_mo3) / (M_mo*C_pmo) + (T_mo2-T_mo3) / tau_mo;
DT_mo4 = ( (1-F_r)*P_cor1*P_cor ) / (M_mo*C_pmo) + (H_fm*A_fm)*(T_f2-T_mo3) / (M_mo*C_pmo) + (T_mo3-T_mo4) / tau_mo;

DT_f3 = (F_r*P_cor1*P_cor) / (M_f*C_pf) + (H_fm*A_fm)*(T_mo5-T_f3) / (M_f *C_pf);
DT_mo5 = ( (1-F_r)*P_cor1*P_cor) / (M_mo*C_pmo) + (H_fm*A_fm) * (T_f3-T_mo5) / (M_mo*C_pmo) + (T_mo4-T_mo5) / tau_mo;
DT_mo6 = ( (1-F_r)*P_cor1*P_cor) / (M_mo*C_pmo) + (H_fm*A_fm) * (T_f3-T_mo5) / (M_mo*C_pmo) + (T_mo5-T_mo6) / tau_mo;

DT_up = (T_mo6-T_up) / tau_up;
DT_hl = (T_up-T_hl) / tau_hl;
DT_lp = (T_cl-T_lp) / tau_lp;
DT_cl = (T_po-T_cl) / tau_cl;


%%%%%% OBLICZENIA DO KONTROLI SYSTEMU REAKTORA
%%%%%zmienne które jeszcze sa wejsciem P,CL,T_fi
POWER_i = 691244.4199;
tau_set = 30;
tau_la1 = 10;
tau_la2 = 5;
tau_le = 80;
tau_rtd = 4;
C_pfw = 1.2181;
K9 = -0.035;
X8 = 1225.85;

T_ave = (T_cl+T_hl) / 2;
DT_hlp = (T_hl-T_hlp) / tau_rtd;
DT_clp = (T_cl-T_clp) / tau_rtd;
T_avep = (T_hlp+T_clp) / 2;

H_st = X8 + (K9*P);
POWER_s= P*C_l*( H_st - (C_pfw*T_fi) );

DT_set = ( 0.19*(POWER_s*100 / POWER_i) + 547 - T_set ) /tau_set;
DT_aves = AUX_co;
DAUX_co = ( T_avep - T_aves - (tau_la1+tau_la2)*AUX_co + tau_le*(DT_clp+DT_hlp) /2 ) / (tau_la1*tau_la2);

%%%%%% STEROWANIE REAKTOREM



e = T_set - T_aves;

React = 0.003375;

 if e >= 5
     dro_ex = (72 * React * 0.00689) / 60;
 elseif e < 5 && e >= 3 
     dro_ex = (React * 0.00689 * (32 * (T_set-T_aves) - 88)) / 60;
 elseif e < 3 && e >= 1 
     dro_ex = (8 * React * 0.00689) / 60;
 elseif abs(e) < 1
     dro_ex = 0;
 elseif e <= -1 && e >= -3 
     dro_ex = (-8 * React * 0.00689) / 60;
 elseif e < -3 && e >= -5
     dro_ex = (React * 0.00689 * (32 * (T_set-T_aves) + 88)) / 60;
 else
     dro_ex = (-72 * React * 0.00689) / 60;
 end
 
 ro_exc= ro_ex*100 / 0.00689 ;
 
%%%%%%%%%%%%%%%%%%%%%%%%%%% REAKTOR

T_f10 = 1488.75;
T_mo10 = 548.303;
T_mo20 = 557.106;
T_f20 = 1506.38;
T_mo30 = 565.909;
T_mo40 = 574.711;
T_f30 = 1523.96;
T_mo50 = 583.514;
T_mo60 = 592.5;

alfa_f = -1.1 * 10^-5;

alfa_c = -2.0 * 10^-4;

RO = ro_ex + alfa_f *( (T_f1-T_f10) + (T_f2-T_f20) + (T_f3-T_f30) ) /3 + alfa_c* ( (T_mo1-T_mo10) + (T_mo2-T_mo20)+ (T_mo3 -T_mo30) + (T_mo4-T_mo40 ) + (T_mo5-T_mo50) + (T_mo6-T_mo60) ) /6;
 
%%%%% ZMIENNE WYJŚCIOWE

dT_f1 = DT_f1;
dT_mo1 = DT_mo1;
dT_mo2 = DT_mo2;
dT_f2 = DT_f2;
dT_mo3 = DT_mo3;
dT_mo4 = DT_mo4;
dT_f3 = DT_f3;
dT_mo5 = DT_mo5;
dT_mo6 = DT_mo6;

dT_up = DT_up;
dT_hl = DT_hl;
dT_lp = DT_lp;
dT_cl = DT_cl;
